simulink model "Acceleration"  (R2019a)
settings: Solver=VariableStepAuto  StartTime=0.0  StopTime=10.0  RelTol=1e-3
undefined symbols (not defined in the file): g, m, my
settings Model: Creator=Frieder Uerlings  LastModifiedBy=Frieder Uerlings

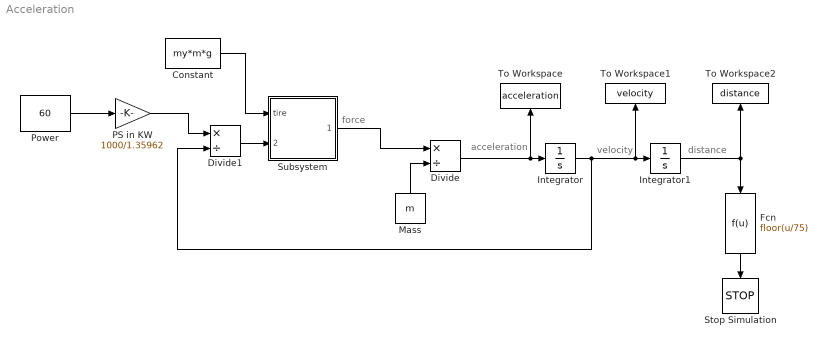
== system Acceleration ==
  note: acceleration
  note: force
  note: distance
  note: velocity
  Constant : Constant  Value=my*m*g
  Divide : Product  Inputs=*/
  Divide1 : Product  Inputs=*/
  Fcn : Fcn  Expr=floor(u/75)
  Integrator : Integrator  InitialCondition=0.01
  Integrator1 : Integrator
  "Mass " : Constant  Value=m  VectorParams1D=off
  "PS in KW " : Gain  Gain=1000/1.35962
  "Power " : Constant  Value=60
  Stop Simulation : Stop
  Subsystem : Subsystem
  To Workspace : ToWorkspace  VariableName=acceleration  SampleTime=-1
  To Workspace1 : ToWorkspace  VariableName=velocity  SampleTime=-1
  To Workspace2 : ToWorkspace  VariableName=distance  SampleTime=-1
  wires:
  "Mass "/1 -> Divide/2
  Divide/1 -> To Workspace/1, Integrator/1
  Integrator/1 -> Divide1/2, To Workspace1/1, Integrator1/1
  Integrator1/1 -> Fcn/1, To Workspace2/1
  "Power "/1 -> "PS in KW "/1
  Fcn/1 -> Stop Simulation/1
  "PS in KW "/1 -> Divide1/1
  Divide1/1 -> Subsystem/2(engine)
  Subsystem/1(max_force) -> Divide/1
  Constant/1 -> Subsystem/1(tire)

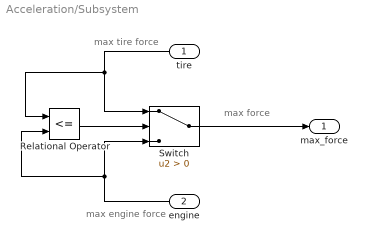
== system Acceleration/Subsystem ==
  note: max force
  note: max tire force
  note: max engine force
  tire : Inport
  engine : Inport  Port=2
  Relational Operator : RelationalOperator  Operator=<=  OutDataTypeStr=boolean  RndMeth=Simplest
  Switch : Switch  Criteria=u2 > Threshold
  max_force : Outport
  wires:
  engine/1 -> Relational Operator/2, Switch/3
  tire/1 -> Relational Operator/1, Switch/1
  Switch/1 -> max_force/1
  Relational Operator/1 -> Switch/2
